simulink model "extractMultiDimFromMessageDemo"  (R2024a)
settings: Solver=FixedStepAuto  StartTime=0.0  StopTime=10.0  RelTol=1e-3
libraries: roshelperlib x6, ros2lib x4
settings Model: DataDictionary=ros2lib.sldd  Creator=cstabile  LastModifiedBy=cstabile

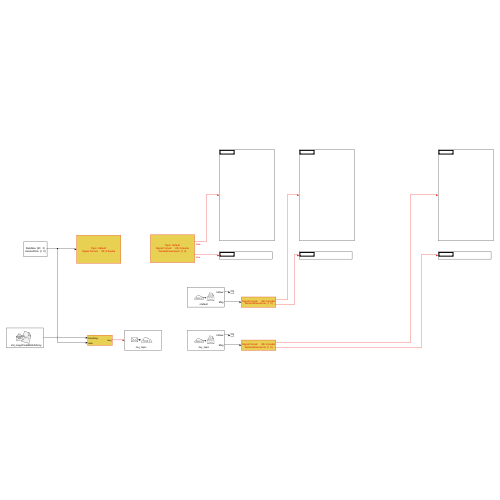
[thumbnail: Simulink's stored preview of the top-level diagram]
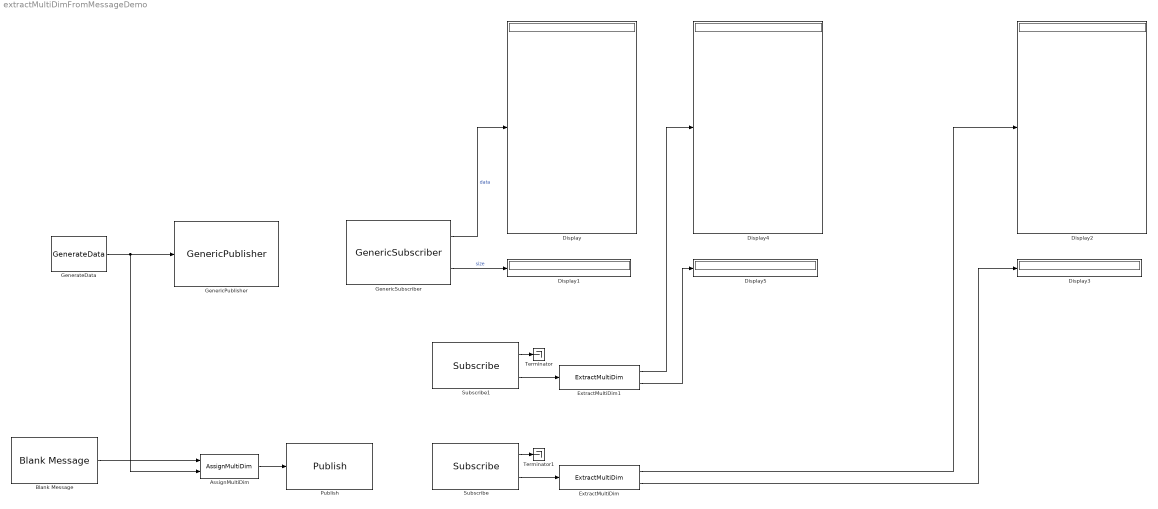
== system extractMultiDimFromMessageDemo ==
  AssignMultiDim : roshelperlib/AssignMultiDim  SystemSampleTime=-1  VariantActivationTime=update diagram  AllowFlexibleInterface=on  Latency=0  AutoFrameSizeCalculation=off
  Blank Message : ros2lib/Blank Message  messageClass=Message  entityType=std_msgs/Float64MultiArray  messageType=std_msgs/Float64MultiArray  SampleTime=inf
  Display{,1..5} (6 alike) : Display
  ExtractMultiDim : roshelperlib/ExtractMultiDim  userDataType=double  dims=[20 3]  isVarsize=on  varsizeDims=[1 0]  returnFixedTF=off
  ExtractMultiDim1 : roshelperlib/ExtractMultiDim  userDataType=double  dims=[20 3]  isVarsize=on  varsizeDims=[1 0]  returnFixedTF=off
  GenerateData : roshelperlib/GenerateData  dataSize=[20 3]  varsizeDims=[1 0]
  GenericPublisher : roshelperlib/GenericPublisher  userDataType=double  dims=[20 3]  topicName='default'  isVarsize=on  varsizeDims=[1 0]
  GenericSubscriber : roshelperlib/GenericSubscriber  userDataType=double  dims=[20 3]  topicName='default'  isVarsize=on  varsizeDims=[1 0]  returnFixedTF=off
  Publish : ros2lib/Publish  topicSource=Specify your own  topic=/my_topic  messageType=std_msgs/Float64MultiArray  QOSHistory=Keep last  QOSDepth=1  QOSReliability=Reliable  QOSDurability=Volatile  QOSDeadline=Inf  QOSLifespan=Inf  QOSLiveliness=Automatic  QOSLeaseDuration=Inf  QOSAvoidROSNamespaceConventions=off
  Subscribe : ros2lib/Subscribe  topicSource=Specify your own  topic=/my_topic  messageType=std_msgs/Float64MultiArray  sampleTime=-1  QOSHistory=Keep last  QOSDepth=1  QOSReliability=Reliable  QOSDurability=Volatile  QOSDeadline=Inf  QOSLifespan=Inf  QOSLiveliness=Automatic  QOSLeaseDuration=Inf  QOSAvoidROSNamespaceConventions=off
  Subscribe1 : ros2lib/Subscribe  topicSource=Specify your own  topic=/default  messageType=std_msgs/Float64MultiArray  sampleTime=-1  QOSHistory=Keep last  QOSDepth=1  QOSReliability=Reliable  QOSDurability=Volatile  QOSDeadline=Inf  QOSLifespan=Inf  QOSLiveliness=Automatic  QOSLeaseDuration=Inf  QOSAvoidROSNamespaceConventions=off
  Terminator : Terminator
  Terminator1 : Terminator
  wires:
  GenerateData/1 -> AssignMultiDim/2, GenericPublisher/1
  GenericSubscriber/1 -> Display/1  "data"
  GenericSubscriber/2 -> Display1/1  "size"
  Blank Message/1 -> AssignMultiDim/1
  AssignMultiDim/1 -> Publish/1
  Subscribe/2 -> ExtractMultiDim/1
  ExtractMultiDim/1 -> Display2/1
  ExtractMultiDim/2 -> Display3/1
  Subscribe1/2 -> ExtractMultiDim1/1
  ExtractMultiDim1/1 -> Display4/1
  ExtractMultiDim1/2 -> Display5/1
  Subscribe1/1 -> Terminator/1
  Subscribe/1 -> Terminator1/1
